simulink model "Inverter"  (R2022a)
settings: Solver=ode1  StartTime=0.0  StopTime=10.0  FixedStep=1e-5  RelTol=1e-3
values from neighbouring files (symbols this model uses):
  Td = 1/fd    (= 0.001)    [PMSMParameters.m]
  VDC = 600    [PMSMParameters.m]
  VP = VDC    (= 600)    [PMSMParameters.m]
libraries: simulink x1
settings Model: Creator=ZinouAb  LastModifiedBy=habayah
settings ModelReferenceCC: EnableRefExpFcnMdlSchedulingChecks=off
settings RTWCC: Description=Generic Real-Time Target

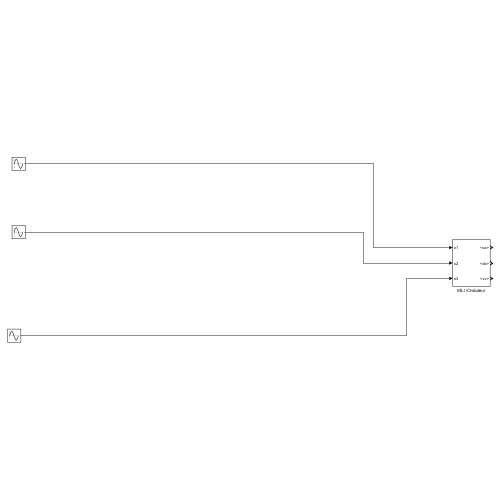
[thumbnail: Simulink's stored preview of the top-level diagram]
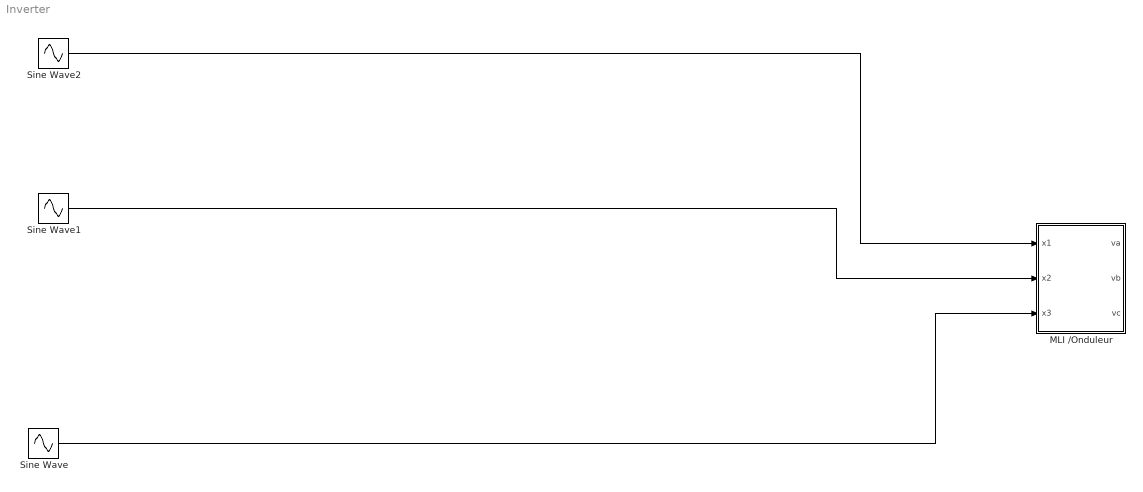
== system Inverter ==
  MLI /Onduleur : Subsystem
  Sine Wave : Sin  Amplitude=220*sqrt(2)  Frequency=2*pi*50  Phase=-4*pi/3  SampleTime=0
  Sine Wave1 : Sin  Amplitude=220*sqrt(2)  Frequency=2*pi*50  Phase=-2*pi/3  SampleTime=0
  Sine Wave2 : Sin  Amplitude=220*sqrt(2)  Frequency=2*pi*50  SampleTime=0
  wires:
  Sine Wave2/1 -> MLI /Onduleur/1(x1)
  Sine Wave1/1 -> MLI /Onduleur/2(x2)
  Sine Wave/1 -> MLI /Onduleur/3(x3)

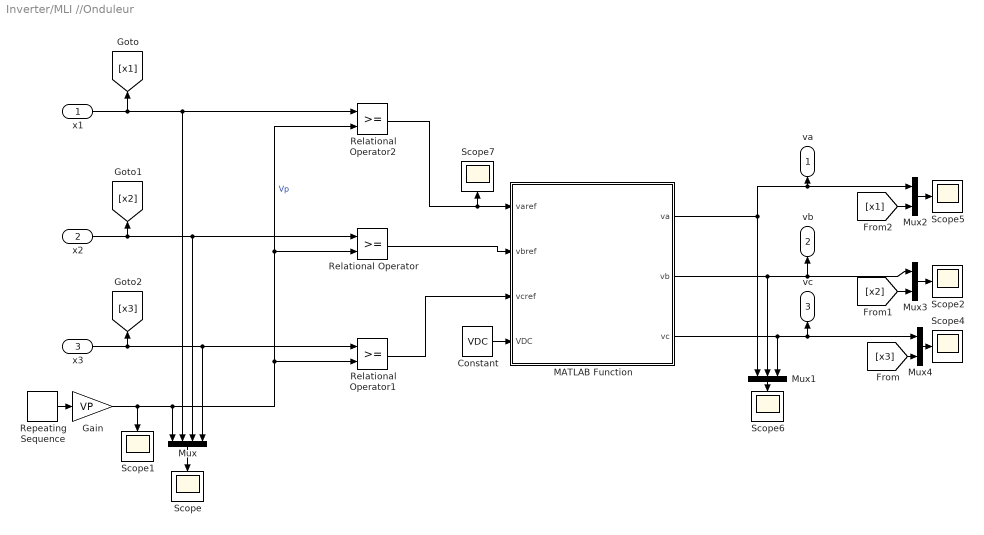
== system Inverter/MLI //Onduleur ==
  x1 : Inport
  x2 : Inport  Port=2
  x3 : Inport  Port=3
  Constant : Constant  Value=VDC
  Gain : Gain  Gain=VP
  MATLAB Function : MATLAB Function  TreatAsAtomicUnit=on
  Mux : Mux
  Mux1 : Mux  Inputs=3
  Mux2 : Mux  Inputs=2
  Mux3 : Mux  Inputs=2
  Mux4 : Mux  Inputs=2
  Relational Operator : RelationalOperator  OutDataTypeStr=boolean  RndMeth=Simplest  InputSameDT=off
  Relational Operator1 : RelationalOperator  OutDataTypeStr=boolean  RndMeth=Simplest  InputSameDT=off
  Relational Operator2 : RelationalOperator  OutDataTypeStr=boolean  RndMeth=Simplest  InputSameDT=off
  Repeating Sequence : simulink/Sources/Repeating Sequence  rep_seq_t=[0 0.5 1].*Td  rep_seq_y=[-1 1 -1]
  Scope{,1..2,4..7} (7 alike) : Scope
  va : Outport
  vb : Outport  Port=2
  vc : Outport  Port=3
  wires:
  Mux/1 -> Scope/1
  Gain/1 -> Scope1/1, Mux/1, Relational Operator1/2, Relational Operator/2, Relational Operator2/2  "Vp"
  Relational Operator/1 -> MATLAB Function/2(vbref)
  Relational Operator1/1 -> MATLAB Function/3(vcref)
  Relational Operator2/1 -> MATLAB Function/1(varef), Scope7/1
  MATLAB Function/1(va) -> va/1, Mux2/1, Mux1/1
  Constant/1 -> MATLAB Function/4(VDC)
  Mux1/1 -> Scope6/1
  Mux2/1 -> Scope5/1
  MATLAB Function/2(vb) -> Mux1/2, vb/1, Mux3/1
  Mux3/1 -> Scope2/1
  MATLAB Function/3(vc) -> Mux1/3, Mux4/1, vc/1
  Mux4/1 -> Scope4/1
  x1/1 -> [x1], Mux/2, Relational Operator2/1
  x2/1 -> Relational Operator/1, Mux/3, [x2]
  x3/1 -> [x3], Mux/4, Relational Operator1/1
  Repeating Sequence/1 -> Gain/1
  [x2] -> Mux3/2
  [x3] -> Mux4/2
  [x1] -> Mux2/2

== matlab function Inverter/MLI //Onduleur/MATLAB Function ==
  data: varef input; vbref input; vcref input; VDC input; va output; vb output; vc output
function [va,vb,vc]= OnduleurOut(varef,vbref,vcref,VDC)
varef=double(varef);
vbref=double(vbref);
vcref=double(vcref);
va=(2*varef-vbref-vcref)*(VDC/3);
vb=(2*vbref-varef-vcref)*(VDC/3);
vc=(2*vcref-vbref-varef)*(VDC/3);
